simulink model "Reifenmodell"  (R2024a)
settings: Solver=VariableStepAuto  StartTime=0.0  StopTime=10.0  RelTol=1e-3
PreLoadFcn:
  | run('Parameter.m')
values from neighbouring files (symbols this model uses):
  g = 9.81    [Model1Sensibilities.m]    (also in Model1numericalPSA.m; Model2Sensibilities.m; Modellvalidierung.m; MotorSens2.m)
  m_last = 0.424    [MotorSens2.m]    (also in Motor_Sensitivitaet.m; Parameter.m = 0.51)
  m_Reifen = 0.038    [MotorSens2.m]    (also in Motor_Sensitivitaet.m; Parameter.m = 0.01; Sensitivitaetsanalyse.m)
  mue = 0.002    [Parameter.m]
  Reifen_Radius = 0.04    [Model1Sensibilities.m]    (also in Model1numericalPSA.m; Model2Sensibilities.m; Modellvalidierung.m; MotorSens2.m)
settings Model: Creator=jakob  LastModifiedBy=jakob

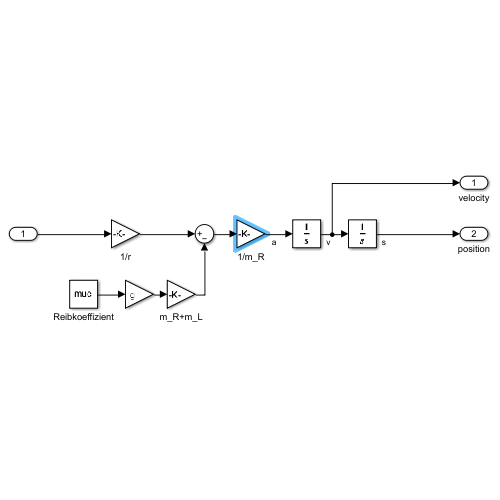
[thumbnail: Simulink's stored preview of the top-level diagram]
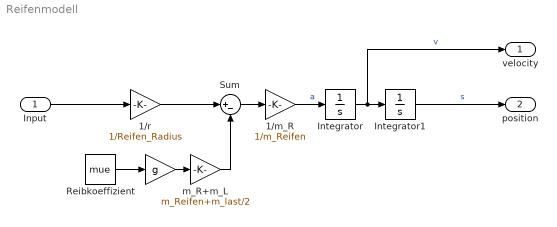
== system Reifenmodell ==
  Input : Inport
  " " : Gain  Gain=g
  1/m_R : Gain  Gain=1/m_Reifen
  1/r : Gain  Gain=1/Reifen_Radius
  Integrator : Integrator  InitialCondition=1
  Integrator1 : Integrator
  Reibkoeffizient : Constant  Value=mue
  Sum : Sum  Inputs=|+-
  m_R+m_L : Gain  Gain=m_Reifen+m_last/2
  velocity : Outport
  position : Outport  Port=2
  wires:
  Reibkoeffizient/1 -> " "/1
  Integrator/1 -> velocity/1, Integrator1/1  "v"
  1/r/1 -> Sum/1
  Input/1 -> 1/r/1
  " "/1 -> m_R+m_L/1
  m_R+m_L/1 -> Sum/2
  Sum/1 -> 1/m_R/1
  1/m_R/1 -> Integrator/1  "a"
  Integrator1/1 -> position/1  "s"
